simulink subsystem "MFTrailerTires"  (R2023a)
settings: Solver=VariableStepAuto  StartTime=0.0  StopTime=10.0  RelTol=1e-3
undefined symbols (not defined in the file): PlntTraInitVertPos, PlntTraNumWhlFrntAxl, PlntTraWhlInitAngVel, PlntTraWhlNomPress
libraries: autolibutils x2, sharedtransform x2, vehdynlibtire x1, vehdynlibtirecommon x1
settings Model: ModifiedByFormat=The MathWorks, Inc.  Creator=The MathWorks, Inc.  LastModifiedBy=The MathWorks, Inc.
settings OptimizationCC: ReuseModelBlockBuffer=off

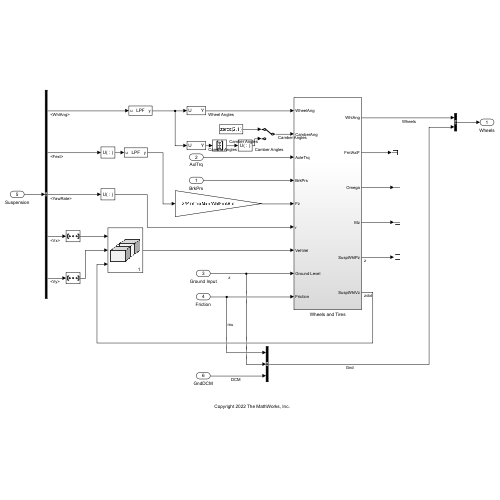
[thumbnail: Simulink's stored preview of the top-level diagram]
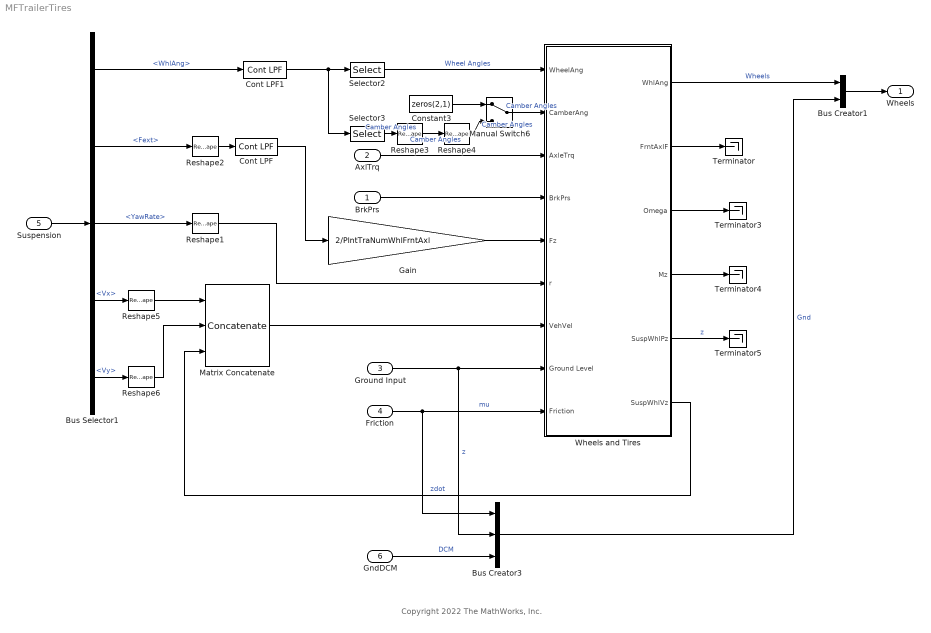
== system MFTrailerTires ==
  note: Copyright 2022 The MathWorks, Inc.
  BrkPrs : Inport
  AxlTrq : Inport  Port=2
  Ground Input : Inport  Port=3
  Friction : Inport  Port=4
  Suspension : Inport  Port=5
  GndDCM : Inport  Port=6
  Bus Creator1 : BusCreator  Inputs=2
  Bus Creator3 : BusCreator  Inputs=3
  Bus Selector1 : BusSelector  OutputSignals=Suspension.WhlAng,Suspension.Fext,Suspension.YawRate,Suspension.Vx,Suspension.Vy
  Constant3 : Constant  Value=zeros(2,1)  SampleTime=-1
  Cont LPF : autolibutils/Cont LPF  wc=100*2*pi  AbsoluteTolerance=auto  aMode=2
  Cont LPF1 : autolibutils/Cont LPF  wc=100*2*pi  AbsoluteTolerance=auto  aMode=2
  Gain : Gain  Gain=2/PlntTraNumWhlFrntAxl
  Manual Switch6 : ManualSwitch
  Matrix Concatenate : Concatenate  NumInputs=3  Mode=Multidimensional array
  Reshape1 : Reshape
  Reshape2 : Reshape
  Reshape3 : Reshape  OutputDimensionality=Column vector (2-D)
  Reshape4 : Reshape
  Reshape5 : Reshape  OutputDimensionality=Row vector (2-D)
  Reshape6 : Reshape  OutputDimensionality=Row vector (2-D)
  Selector2 : Selector  NumberOfDimensions=2  InputPortWidth=3  IndexOptions=Index vector (dialog),Select all  Indices=3,1  OutputSizes=1,1
  Selector3 : Selector  NumberOfDimensions=2  InputPortWidth=3  IndexOptions=Index vector (dialog),Select all  Indices=1,1  OutputSizes=1,1
  Terminator{,3..5} (4 alike) : Terminator
  Wheels and Tires : Subsystem  VariantControl=0
  Wheels : Outport  VectorParamsAs1DForOutWhenUnconnected=off
  wires:
  Ground Input/1 -> Wheels and Tires/8(Ground Level), Bus Creator3/2  "z"
  GndDCM/1 -> Bus Creator3/3  "DCM"
  Friction/1 -> Bus Creator3/1, Wheels and Tires/9(Friction)  "mu"
  Bus Creator3/1 -> Bus Creator1/2  "Gnd"
  Bus Creator1/1 -> Wheels/1
  Selector3/1 -> Reshape3/1  "Camber Angles"
  Reshape2/1 -> Cont LPF/1
  Reshape1/1 -> Wheels and Tires/6(r)
  Cont LPF/1 -> Gain/1
  BrkPrs/1 -> Wheels and Tires/4(BrkPrs)
  Cont LPF1/1 -> Selector3/1, Selector2/1
  Wheels and Tires/6(SuspWhlVz) -> Matrix Concatenate/3  "zdot"
  Bus Selector1/1 -> Cont LPF1/1  "<WhlAng>"
  Manual Switch6/1 -> Wheels and Tires/2(CamberAng)  "Camber Angles"
  Bus Selector1/5 -> Reshape6/1  "<Vy>"
  Bus Selector1/4 -> Reshape5/1  "<Vx>"
  Reshape3/1 -> Reshape4/1  "Camber Angles"
  Suspension/1 -> Bus Selector1/1
  Bus Selector1/3 -> Reshape1/1  "<YawRate>"
  Wheels and Tires/3(Omega) -> Terminator3/1
  Constant3/1 -> Manual Switch6/1
  Wheels and Tires/4(Mz) -> Terminator4/1
  Wheels and Tires/5(SuspWhlPz) -> Terminator5/1  "z"
  Bus Selector1/2 -> Reshape2/1  "<Fext>"
  AxlTrq/1 -> Wheels and Tires/3(AxleTrq)
  Reshape4/1 -> Manual Switch6/2  "Camber Angles"
  Wheels and Tires/1(WhlAng) -> Bus Creator1/1  "Wheels"
  Gain/1 -> Wheels and Tires/5(Fz)
  Selector2/1 -> Wheels and Tires/1(WheelAng)  "Wheel Angles"
  Matrix Concatenate/1 -> Wheels and Tires/7(VehVel)
  Wheels and Tires/2(FrntAxlF) -> Terminator/1
  Reshape5/1 -> Matrix Concatenate/1
  Reshape6/1 -> Matrix Concatenate/2

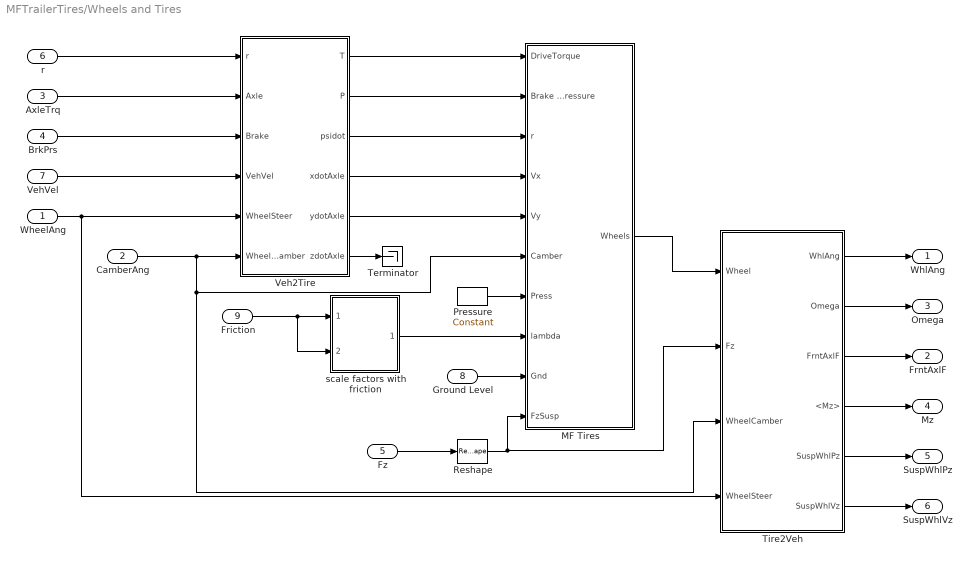
== system MFTrailerTires/Wheels and Tires ==
  WheelAng : Inport
  CamberAng : Inport  Port=2  Unit=rad
  AxleTrq : Inport  Port=3
  BrkPrs : Inport  Port=4
  Fz : Inport  Port=5  Unit=N
  r : Inport  Port=6
  VehVel : Inport  Port=7
  Ground Level : Inport  Port=8
  Friction : Inport  Port=9  Unit=1
  MF Tires : Subsystem  VariantControl=0
  Pressure : vehdynlibtirecommon/Constant  const=PlntTraWhlNomPress  numWheels=2
  Reshape : Reshape
  Terminator : Terminator
  Tire2Veh : Subsystem
  Veh2Tire : Subsystem
  scale factors with friction : Subsystem  mask{numWheels=6}
      mask prompts: numWheels "Number of wheels"
  WhlAng : Outport  VectorParamsAs1DForOutWhenUnconnected=off
  FrntAxlF : Outport  Port=2  Unit=N  VectorParamsAs1DForOutWhenUnconnected=off
  Omega : Outport  Port=3  VectorParamsAs1DForOutWhenUnconnected=off
  Mz : Outport  Port=4  Unit=N*m  VectorParamsAs1DForOutWhenUnconnected=off
  SuspWhlPz : Outport  Port=5  VectorParamsAs1DForOutWhenUnconnected=off
  SuspWhlVz : Outport  Port=6  VectorParamsAs1DForOutWhenUnconnected=off
  wires:
  Reshape/1 -> MF Tires/10(FzSusp), Tire2Veh/2(Fz)
  Ground Level/1 -> MF Tires/9(Gnd)
  Pressure/1 -> MF Tires/7(Press)
  scale factors with friction/1(lambdas) -> MF Tires/8(lambda)
  Fz/1 -> Reshape/1
  AxleTrq/1 -> Veh2Tire/2(Axle)
  BrkPrs/1 -> Veh2Tire/3(Brake)
  VehVel/1 -> Veh2Tire/4(VehVel)
  Veh2Tire/1(T) -> MF Tires/1(DriveTorque)
  Veh2Tire/2(P) -> MF Tires/2(Brake Pressure)
  Veh2Tire/4(xdotAxle) -> MF Tires/4(Vx)
  Veh2Tire/5(ydotAxle) -> MF Tires/5(Vy)
  Veh2Tire/3(psidot) -> MF Tires/3(r)
  MF Tires/1(Wheels) -> Tire2Veh/1(Wheel)
  WheelAng/1 -> Veh2Tire/5(WheelSteer), Tire2Veh/4(WheelSteer)
  Tire2Veh/2(Omega) -> Omega/1
  Tire2Veh/3(FrntAxlF) -> FrntAxlF/1
  Tire2Veh/4(<Mz>) -> Mz/1
  Friction/1 -> scale factors with friction/1(lamda_mu_x), scale factors with friction/2(lamda_mu_y)
  r/1 -> Veh2Tire/1(r)
  Veh2Tire/6(zdotAxle) -> Terminator/1
  Tire2Veh/5(SuspWhlPz) -> SuspWhlPz/1
  Tire2Veh/6(SuspWhlVz) -> SuspWhlVz/1
  CamberAng/1 -> MF Tires/6(Camber), Tire2Veh/3(WheelCamber), Veh2Tire/6(WheelCamber)
  Tire2Veh/1(WhlAng) -> WhlAng/1

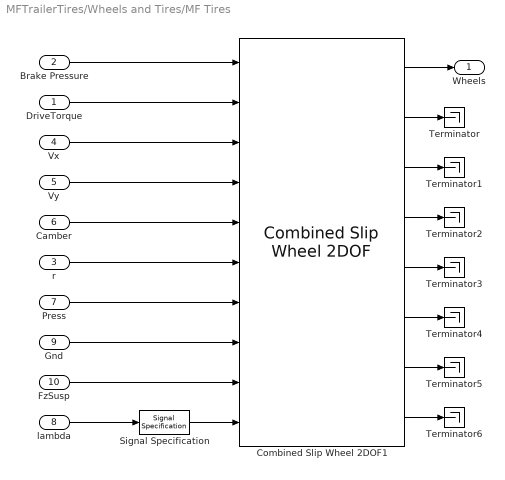
== system MFTrailerTires/Wheels and Tires/MF Tires ==
  DriveTorque : Inport
  Brake Pressure : Inport  Port=2
  r : Inport  Port=3
  Vx : Inport  Port=4
  Vy : Inport  Port=5
  Camber : Inport  Port=6
  Press : Inport  Port=7  Unit=Pa
  lambda : Inport  Port=8  Unit=1
  Gnd : Inport  Port=9
  FzSusp : Inport  Port=10
  Combined Slip Wheel 2DOF1 : vehdynlibtire/Combined Slip Wheel 2DOF  tireType=Mid-size passenger car 235/45R18  BrakeType=Disc  vertType=Magic Formula  plySteer=off  turnslip=off  mu_static=PlntTraBrkStcFricCffFrnt  mu_kinetic=PlntTraBrkKinFricCffFrnt  disk_abore=PlntTraBrkActrBoreFrnt  Rm=PlntTraBrkPadMeanRadiusFrnt  num_pads=PlntTraBrkNumPadsFrnt  drum_abore=0.0508  drum_a=0.123  drum_c=0.212  drum_r=0.15  drum_theta1=0  drum_theta2=126  brake_p_bpt=[1 11.4736842105263 21.9473684210526 32.4210526315789 42.8947368421053 53.3684210526316 63.8421052631579 74.3157894736842 84.7894736842105 95.2631578947368 105.736842105263 116.210526315789 126.684210526316 137.157894736842 147.631578947368 158.105263157895 168.578947368421 179.052631578947 189.526315789474 200]  brake_n_bpt=[0 52.6315789473684 105.263157894737 157.894736842105 210.526315789474 263.157894736842 315.789473684211 368.421052631579 421.052631578947 473.684210526316 526.315789473684 578.947368421053 631.578947368421 684.210526315789 736.842105263158 789.473684210526 842.105263157895 894.736842105263 947.368421052632 1000]  f_brake_t=[43.4900602404453 42.5056030554862 41.5350898940194 40.5780454442085 39.6340111501808 38.7025443887544 37.7832176914519 36.8756180088306 35.9793460143796 35.0940154454303 34.2192524787115 33.3546951383474 32.4999927342521 31.6548053290159 30.8188032315107 29.991666515561 29.1730845621415 28.362755623661 27.5603864089927 26.765691687993;498.991217495636 487.695866636631 476.560505099801 465.579679307235 454.748127933653 444.060772460445 433.51270824929 423.099196101319 412.81565427025 402.657650900201 392.620896861006 382.701238955775 372.894653477208 363.197240090814 353.605216024701 344.114910546964 334.722759712992 325.425301366216 316.219170376863 307.10109410434;954.492374750826 932.886130217776 911.585920305583 890.581313170261 869.862244717126 849.419000532136 829.242198807128 809.322774193808 789.651962526121 770.221286354971 751.0225412433 732.047782773203 713.289314220164 694.739674852612 676.391628817892 658.238154578366 640.272434863842 622.48784710877 604.877954344734 587.436496520688;1409.99353200602 1378.07639379892 1346.61133551136 1315.58294703329 1284.9763615006 1254.77722860383 1224.97168936497 1195.5463522863 1166.48827078199 1137.78492180974 1109.42418562559 1081.39432659063 1053.68397496312 1026.28210961441 999.178041611083 972.361398609768 945.822110014692 919.550392851325 893.536738312604 867.771898937035;1865.49468926121 1823.26665738007 1781.63675071715 1740.58458089631 1700.09047828407 1660.13545667552 1620.7011799228 1581.76993037878 1543.32457903786 1505.34855726451 1467.82583000789 1430.74087040806 1394.07863570608 1357.82454437621 1321.96445440427 1286.48464264117 1251.37178516554 1216.61293859388 1182.19552228048 1148.10730135338;2320.9958465164 2268.45692096121 2216.66216592293 2165.58621475934 2115.20459506754 2065.49368474721 2016.43067048064 1967.99350847127 1920.16088729373 1872.91219271928 1826.22747439018 1780.08741422549 1734.47329644903 1689.36697913801 1644.75086719747 1600.60788667257 1556.92146031639 1513.67548433643 1470.85430624835 1428.44270376973;2776.49700377159 2713.64718454235 2651.68758112871 2590.58784862237 2530.31871185102 2470.8519128189 2412.16016103848 2354.21708656376 2296.9971955496 2240.47582817405 2184.62911877248 2129.43395804292 2074.86795719199 2020.9094138998 1967.53727999066 1914.73113070398 1862.47113546724 1810.73803007899 1759.51309021622 1708.77810618608;3231.99816102678 3158.8374481235 3086.71299633449 3015.58948248539 2945.43282863449 2876.21014089059 2807.88965159632 2740.44066465625 2673.83350380547 2608.03946362882 2543.03076315477 2478.78050186034 2415.26261793494 2352.4518486616 2290.32369278385 2228.85437473538 2168.02081061809 2107.80057582154 2048.17187418409 1989.11350860242;3687.49931828197 3604.02771170464 3521.73841154027 3440.59111634842 3360.54694541796 3281.56836896228 3203.61914215416 3126.66424274874 3050.66981206134 2975.60309908359 2901.43240753707 2828.12704567777 2755.6572786779 2683.9942834234 2613.11010557704 2542.97761876678 2473.57048576894 2404.8631215641 2336.83065815196 2269.44891101877;4143.00047553716 4049.21797528579 3956.76382674606 3865.59275021144 3775.66106220143 3686.92659703397 3599.34863271199 3512.88782084123 3427.50612031721 3343.16673453836 3259.83405191936 3177.4735894952 3096.05193942085 3015.5367181852 2935.89651837023 2857.10086279818 2779.12016091979 2701.92566730665 2625.48944211983 2549.78431343512;4598.50163279235 4494.40823886693 4391.78924195184 4290.59438407447 4190.77517898491 4092.28482510566 3995.07812326983 3899.11139893372 3804.34242857308 3710.73036999313 3618.23569630166 3526.82013331263 3436.44660016381 3347.079152947 3258.68293116342 3171.22410682959 3084.66983607064 2998.98821304921 2914.1482260877 2830.11971585147;5054.00279004754 4939.59850244808 4826.81465715762 4715.59601793749 4605.88929576838 4497.64305317735 4390.80761382767 4285.3349770262 4181.17873682896 4078.2940054479 3976.63734068395 3876.16667713006 3776.84126090677 3678.62158770879 3581.46934395661 3485.34735086099 ...(+2764 chars)]  tireParamSet=C:\SimTemp\GCAPS_Goodyear_MarathonRSA_295_75_R22.5_8.25J_141L_MF62turnslip_CA_YL_MAY042020.tir  PRESMAX=PlntTraWhlMaxPress  PRESMIN=PlntTraWhlMinPress  FZMAX=PlntTraWhlMaxFz  FZMIN=PlntTraWhlMinFz  VXLOW=PlntTraWhlVelTolLowVel  KPUMAX=PlntTraWhlMaxSlipRatio  KPUMIN=PlntTraWhlMinSlipRatio  ALPMAX=PlntTraWhlMaxSlipAngle  ALPMIN=PlntTraWhlMinSlipAngle  CAMMAX=PlntTraWhlMaxCmbr  CAMMIN=PlntTraWhlMinCmbr  LONGVL=PlntTraWhlLongSpd  FxRelFreqLwrLim=200*pi  FyRelFreqLwrLim=200*pi  MyRelFreqLwrLim=100*pi  omegao=[PlntTraWhlInitAngVel PlntTraWhlInitAngVel]  br=PlntTraWhlDampCoeff  UNLOADED_RADIUS=PlntTraWhlUnldRadius  NOMPRES=PlntTraWhlNomPress  FNOMIN=PlntTraWhlNomNorlForce  WIDTH=PlntTraWhlWidth  RIM_RADIUS=PlntTraWhlRimRadius  MASS=PlntTraWhlMass  IYY=PlntTraWhlInertia  GRAVITY=-9.81  zo=-PlntTraInitVertPos  zdoto=0  BREFF=8.392  DREFF=0.03576  FREFF=0.4661  Q_RE0=1.0016  Q_V1=0.0003732  Q_V2=0.02362  Q_FZ1=0  Q_FZ2=133.78  Q_FZ3=0  Q_FCX=0  Q_FCY=0  Q_FCY2=0  PFZ1=0  VERTICAL_STIFFNESS=910293.6  VERTICAL_DAMPING=PlntTraWhlVertDampCoeff  BOTTOM_OFFST=0.01  BOTTOM_STIFF=2000000  LONGITUDINAL_STIFFNESS=658043.3  LATERAL_STIFFNESS=334950.6  PCFX1=-0.05681  PCFX2=0  PCFX3=0  PCFY1=-0.012727  PCFY2=0  PCFY3=0  Q_RA1=1  Q_RA2=0.167  Q_RB1=1.4176  Q_RB2=-3.104  PCX1=1.6344  PDX1=0.8142  PDX2=-0.16106  PDX3=0  PEX1=0.14852  PEX2=0.10924  PEX3=0  PEX4=0.6315  PKX1=12.27  PKX2=0.07478  PKX3=-0.02593  PHX1=-0.002517  PHX2=-5.505e-05  PVX1=0.018635  PVX2=0.004217  PPX1=0  PPX2=0  PPX3=0  PPX4=0  RBX1=14.568  RBX2=26.13  RBX3=0  RCX1=0.67  REX1=-10  REX2=1.2903  RHX1=0.006853  QSX1=0.0015863  QSX2=0.7911  QSX3=0.005838  QSX4=0.6123  QSX5=1.0173  QSX6=1.0795  QSX7=-1  QSX8=-0.07876  QSX9=1.5937  QSX10=0.20124  QSX11=7.712  QSX12=0  QSX13=0  QSX14=0  PPMX1=0  PCY1=1.7918  PDY1=0.8339  PDY2=-0.16352  PDY3=0  PEY1=0.3527  PEY2=-0.4847  PEY3=-0.04566  PEY4=-0.8786  PEY5=0  PKY1=-25.044  PKY2=5  PKY3=-0.35276  PKY4=1.397  PKY5=0  PKY6=-0.14207  PKY7=0.2761  PHY1=0.004573  PHY2=0.0011903  PVY1=0.012717  PVY2=-0.005622  PVY3=-0.5051  PVY4=-0.20847  PPY1=0  PPY2=0  PPY3=0  PPY4=0  PPY5=0  RBY1=11.94  RBY2=7.527  RBY3=-0.04993  RBY4=0  RCY1=1.011  REY1=0.5603  REY2=-0.015398  RHY1=0.003565  RHY2=-0.004565  RVY1=-0.02114  RVY2=0.00636  RVY3=0.5299  RVY4=15  RVY5=2.2  RVY6=6.517  QSY1=0.01  QSY2=0  QSY3=0.0004  QSY4=4e-05  QSY5=0  QSY6=0  QSY7=0.85  QSY8=-0.4  QBZ1=5  QBZ2=0.11227  QBZ3=0  QBZ4=0.3959  QBZ5=0.6941  QBZ6=0  QBZ9=7.076  QBZ10=0  QCZ1=1.6  QDZ1=0.05489  QDZ2=-0.014706  QDZ3=0.23333  QDZ4=0  QDZ6=-0.002125  QDZ7=0.0019598  QDZ8=-0.05395  QDZ9=0.011456  QDZ10=0  QDZ11=0  QEZ1=-0.2972  QEZ2=0.0005504  QEZ3=0  QEZ4=0.8904  QEZ5=-15  QHZ1=0.009102  QHZ2=-0.0012268  QHZ3=0.24217  QHZ4=-0.2619  PPZ1=0  PPZ2=0  SSZ1=-0.011962  SSZ2=0.01055  SSZ3=0.885  SSZ4=-0.3521  PDXP1=0.4  PDXP2=0  PDXP3=0  PKYP1=0.1  PDYP1=0.4  PDYP2=0  PDYP3=0  PDYP4=0  PHYP1=1  PHYP2=0.15  PHYP3=0  PHYP4=-4  PECP1=0.68093  PECP2=1.5779e-08  QDTP1=5.6762  QCRP1=0.11047  QCRP2=0.1  QBRP1=0.10576  QDRP1=1  QDRP2=0  aMode=2
      settings: SourceProductName=Vehicle Dynamics Blockset
  Signal Specification : SignalSpecification  Unit=1
  Terminator{,1..6} (7 alike) : Terminator
  Wheels : Outport  VectorParamsAs1DForOutWhenUnconnected=off
  wires:
  FzSusp/1 -> Combined Slip Wheel 2DOF1/9
  Combined Slip Wheel 2DOF1/2 -> Terminator/1
  Gnd/1 -> Combined Slip Wheel 2DOF1/8
  Combined Slip Wheel 2DOF1/1 -> Wheels/1
  Brake Pressure/1 -> Combined Slip Wheel 2DOF1/1
  DriveTorque/1 -> Combined Slip Wheel 2DOF1/2
  Press/1 -> Combined Slip Wheel 2DOF1/7
  r/1 -> Combined Slip Wheel 2DOF1/6
  Camber/1 -> Combined Slip Wheel 2DOF1/5
  lambda/1 -> Signal Specification/1
  Vx/1 -> Combined Slip Wheel 2DOF1/3
  Vy/1 -> Combined Slip Wheel 2DOF1/4
  Signal Specification/1 -> Combined Slip Wheel 2DOF1/10
  Combined Slip Wheel 2DOF1/3 -> Terminator1/1
  Combined Slip Wheel 2DOF1/4 -> Terminator2/1
  Combined Slip Wheel 2DOF1/7 -> Terminator5/1
  Combined Slip Wheel 2DOF1/6 -> Terminator4/1
  Combined Slip Wheel 2DOF1/5 -> Terminator3/1
  Combined Slip Wheel 2DOF1/8 -> Terminator6/1

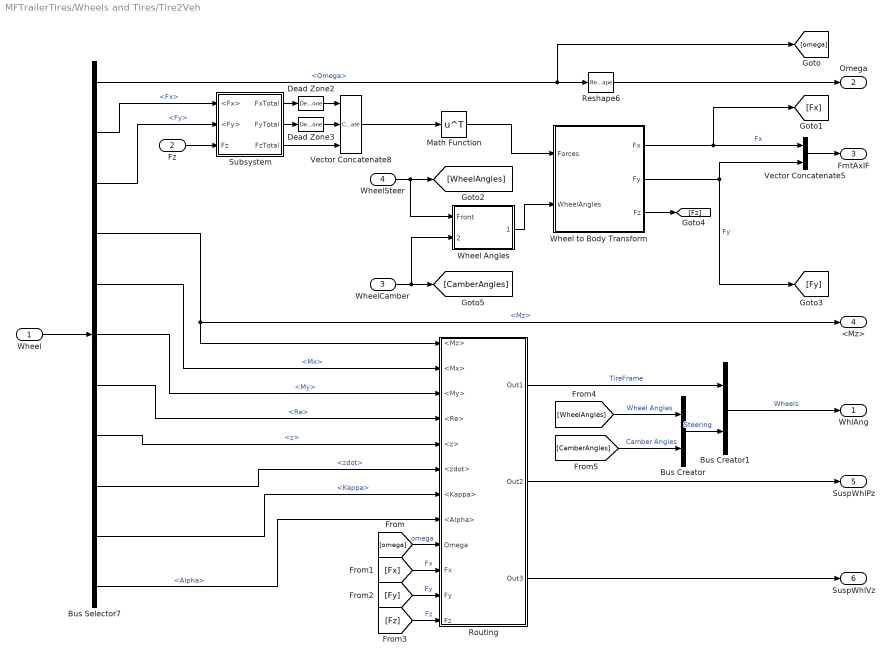
== system MFTrailerTires/Wheels and Tires/Tire2Veh ==
  Wheel : Inport
  Fz : Inport  Port=2
  WheelCamber : Inport  Port=3
  WheelSteer : Inport  Port=4
  Bus Creator : BusCreator  Inputs=2
  Bus Creator1 : BusCreator  Inputs=2
  Bus Selector7 : BusSelector  OutputSignals=Omega,Fx,Fy,Mz,Mx,My,Re,z,zdot,Kappa,Alpha
  Dead Zone2 : DeadZone  LowerValue=-5  UpperValue=5  ZeroCross=off
  Dead Zone3 : DeadZone  LowerValue=-10  UpperValue=10  ZeroCross=off
  Math Function : Math  Operator=transpose  SignedPower=on
  Reshape6 : Reshape  OutputDimensionality=Customize  OutputDimensions=[2,1]
  Routing : Subsystem
  Subsystem : Subsystem
  Vector Concatenate5 : Concatenate  Mode=Multidimensional array  ConcatenateDimension=2
  Vector Concatenate8 : Concatenate  NumInputs=3  Mode=Multidimensional array  ConcatenateDimension=2
  Wheel Angles : Subsystem
  Wheel to Body Transform : Subsystem
  WhlAng : Outport  VectorParamsAs1DForOutWhenUnconnected=off
  Omega : Outport  Port=2  VectorParamsAs1DForOutWhenUnconnected=off
  FrntAxlF : Outport  Port=3  VectorParamsAs1DForOutWhenUnconnected=off
  <Mz> : Outport  Port=4  VectorParamsAs1DForOutWhenUnconnected=off
  SuspWhlPz : Outport  Port=5  VectorParamsAs1DForOutWhenUnconnected=off
  SuspWhlVz : Outport  Port=6  VectorParamsAs1DForOutWhenUnconnected=off
  wires:
  Dead Zone3/1 -> Vector Concatenate8/2
  Dead Zone2/1 -> Vector Concatenate8/1
  Subsystem/3(FzTotal) -> Vector Concatenate8/3
  Subsystem/2(FyTotal) -> Dead Zone3/1
  Subsystem/1(FxTotal) -> Dead Zone2/1
  Fz/1 -> Subsystem/3(Fz)
  Bus Selector7/3 -> Subsystem/2(<Fy>)  "<Fy>"
  Bus Selector7/2 -> Subsystem/1(<Fx>)  "<Fx>"
  Vector Concatenate8/1 -> Math Function/1
  Math Function/1 -> Wheel to Body Transform/1(Forces)
  Wheel to Body Transform/1(Fx) -> Vector Concatenate5/1, [Fx]  "Fx"
  Vector Concatenate5/1 -> FrntAxlF/1
  Wheel/1 -> Bus Selector7/1
  Reshape6/1 -> Omega/1
  Wheel to Body Transform/2(Fy) -> Vector Concatenate5/2, [Fy]  "Fy"
  Wheel Angles/1(Vehicle) -> Wheel to Body Transform/2(WheelAngles)
  Bus Selector7/1 -> [omega], Reshape6/1  "<Omega>"
  WheelSteer/1 -> Wheel Angles/1(Front), [WheelAngles]
  Bus Selector7/4 -> <Mz>/1, Routing/1(<Mz>)  "<Mz>"
  Wheel to Body Transform/3(Fz) -> [Fz]
  WheelCamber/1 -> Wheel Angles/2(Camber), [CamberAngles]
  Bus Selector7/5 -> Routing/2(<Mx>)  "<Mx>"
  Bus Selector7/6 -> Routing/3(<My>)  "<My>"
  Bus Selector7/7 -> Routing/4(<Re>)  "<Re>"
  [omega] -> Routing/9(Omega)  "omega"
  [Fx] -> Routing/10(Fx)  "Fx"
  Bus Selector7/8 -> Routing/5(<z>)  "<z>"
  [Fy] -> Routing/11(Fy)  "Fy"
  [Fz] -> Routing/12(Fz)  "Fz"
  Bus Selector7/9 -> Routing/6(<zdot>)  "<zdot>"
  Bus Selector7/10 -> Routing/7(<Kappa>)  "<Kappa>"
  Routing/2(Out2) -> SuspWhlPz/1
  Routing/3(Out3) -> SuspWhlVz/1
  [WheelAngles] -> Bus Creator/1  "Wheel Angles"
  Bus Creator1/1 -> WhlAng/1  "Wheels"
  Routing/1(Out1) -> Bus Creator1/1  "TireFrame"
  [CamberAngles] -> Bus Creator/2  "Camber Angles"
  Bus Creator/1 -> Bus Creator1/2  "Steering"
  Bus Selector7/11 -> Routing/8(<Alpha>)  "<Alpha>"

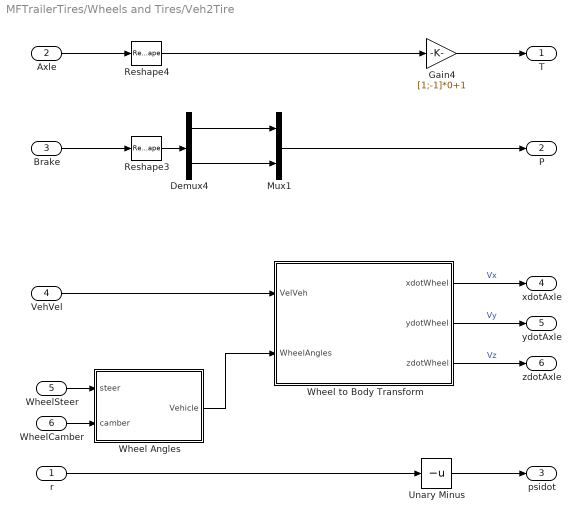
== system MFTrailerTires/Wheels and Tires/Veh2Tire ==
  r : Inport
  Axle : Inport  Port=2
  Brake : Inport  Port=3
  VehVel : Inport  Port=4
  WheelSteer : Inport  Port=5
  WheelCamber : Inport  Port=6
  Demux4 : Demux  Outputs=2
  Gain4 : Gain  Gain=[1;-1]*0+1
  Mux1 : Mux  Inputs=2
  Reshape3 : Reshape
  Reshape4 : Reshape
  Unary Minus : UnaryMinus
  Wheel Angles : Subsystem
  Wheel to Body Transform : Subsystem
  T : Outport  Unit=N*m  VectorParamsAs1DForOutWhenUnconnected=off
  P : Outport  Port=2  Unit=Pa  VectorParamsAs1DForOutWhenUnconnected=off
  psidot : Outport  Port=3  Unit=rad/s  VectorParamsAs1DForOutWhenUnconnected=off
  xdotAxle : Outport  Port=4  Unit=m/s  VectorParamsAs1DForOutWhenUnconnected=off
  ydotAxle : Outport  Port=5  Unit=m/s  VectorParamsAs1DForOutWhenUnconnected=off
  zdotAxle : Outport  Port=6  Unit=m/s  VectorParamsAs1DForOutWhenUnconnected=off
  wires:
  Demux4/2 -> Mux1/2
  Demux4/1 -> Mux1/1
  Brake/1 -> Reshape3/1
  Axle/1 -> Reshape4/1
  Wheel to Body Transform/1(xdotWheel) -> xdotAxle/1  "Vx"
  Wheel to Body Transform/2(ydotWheel) -> ydotAxle/1  "Vy"
  WheelSteer/1 -> Wheel Angles/1(steer)
  Mux1/1 -> P/1
  r/1 -> Unary Minus/1
  Reshape3/1 -> Demux4/1
  Gain4/1 -> T/1
  Reshape4/1 -> Gain4/1
  VehVel/1 -> Wheel to Body Transform/1(VelVeh)
  Wheel to Body Transform/3(zdotWheel) -> zdotAxle/1  "Vz"
  WheelCamber/1 -> Wheel Angles/2(camber)
  Unary Minus/1 -> psidot/1
  Wheel Angles/1(Vehicle) -> Wheel to Body Transform/2(WheelAngles)

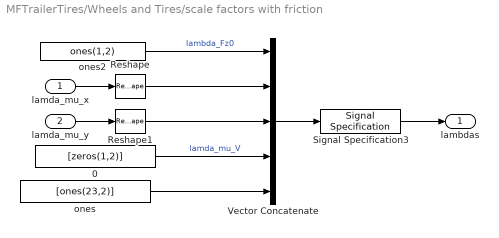
== system MFTrailerTires/Wheels and Tires/scale factors with friction ==
  lamda_mu_x : Inport
  lamda_mu_y : Inport  Port=2
  0 : Constant  Value=[zeros(1,2)]  VectorParams1D=off
  Reshape : Reshape  OutputDimensionality=Row vector (2-D)  OutputDimensions=[1,numWheels]
  Reshape1 : Reshape  OutputDimensionality=Row vector (2-D)  OutputDimensions=[1,numWheels]
  Signal Specification3 : SignalSpecification  Unit=1
  Vector Concatenate : Concatenate  NumInputs=5  Mode=Multidimensional array
  ones : Constant  Value=[ones(23,2)]  VectorParams1D=off
  ones2 : Constant  Value=ones(1,2)  VectorParams1D=off
  lambdas : Outport  Unit=1  VectorParamsAs1DForOutWhenUnconnected=off
  wires:
  Signal Specification3/1 -> lambdas/1
  Reshape/1 -> Vector Concatenate/2
  Reshape1/1 -> Vector Concatenate/3
  0/1 -> Vector Concatenate/4  "lamda_mu_V"
  ones/1 -> Vector Concatenate/5
  Vector Concatenate/1 -> Signal Specification3/1
  ones2/1 -> Vector Concatenate/1  "lambda_Fz0"
  lamda_mu_x/1 -> Reshape/1
  lamda_mu_y/1 -> Reshape1/1

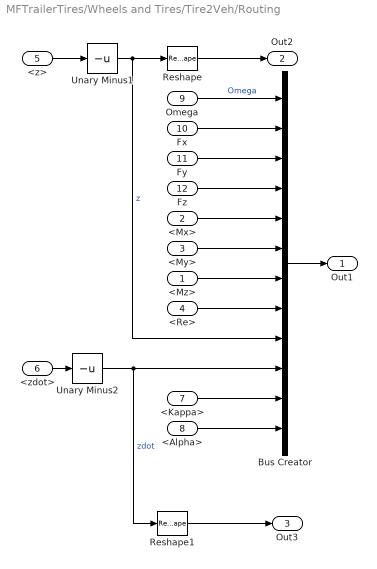
== system MFTrailerTires/Wheels and Tires/Tire2Veh/Routing ==
  <Mz> : Inport
  <Mx> : Inport  Port=2
  <My> : Inport  Port=3
  <Re> : Inport  Port=4
  <z> : Inport  Port=5
  <zdot> : Inport  Port=6
  <Kappa> : Inport  Port=7
  <Alpha> : Inport  Port=8
  Omega : Inport  Port=9
  Fx : Inport  Port=10
  Fy : Inport  Port=11
  Fz : Inport  Port=12
  Bus Creator : BusCreator  Inputs=12
  Reshape : Reshape  OutputDimensionality=Row vector (2-D)
  Reshape1 : Reshape  OutputDimensionality=Row vector (2-D)
  Unary Minus1 : UnaryMinus
  Unary Minus2 : UnaryMinus
  Out1 : Outport  VectorParamsAs1DForOutWhenUnconnected=off
  Out2 : Outport  Port=2  VectorParamsAs1DForOutWhenUnconnected=off
  Out3 : Outport  Port=3  VectorParamsAs1DForOutWhenUnconnected=off
  wires:
  <Re>/1 -> Bus Creator/8
  Unary Minus1/1 -> Reshape/1, Bus Creator/9  "z"
  Fz/1 -> Bus Creator/4
  <zdot>/1 -> Unary Minus2/1
  <Mz>/1 -> Bus Creator/7
  Unary Minus2/1 -> Reshape1/1, Bus Creator/10  "zdot"
  <z>/1 -> Unary Minus1/1
  Bus Creator/1 -> Out1/1
  Fy/1 -> Bus Creator/3
  Omega/1 -> Bus Creator/1  "Omega"
  Fx/1 -> Bus Creator/2
  Reshape1/1 -> Out3/1
  <Kappa>/1 -> Bus Creator/11
  Reshape/1 -> Out2/1
  <Mx>/1 -> Bus Creator/5
  <My>/1 -> Bus Creator/6
  <Alpha>/1 -> Bus Creator/12

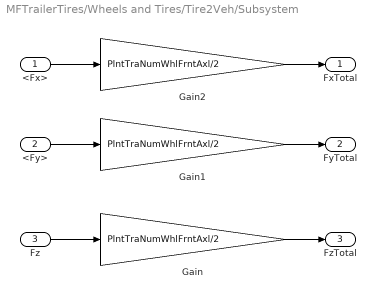
== system MFTrailerTires/Wheels and Tires/Tire2Veh/Subsystem ==
  <Fx> : Inport
  <Fy> : Inport  Port=2
  Fz : Inport  Port=3
  Gain : Gain  Gain=PlntTraNumWhlFrntAxl/2
  Gain1 : Gain  Gain=PlntTraNumWhlFrntAxl/2
  Gain2 : Gain  Gain=PlntTraNumWhlFrntAxl/2
  FxTotal : Outport
  FyTotal : Outport  Port=2
  FzTotal : Outport  Port=3
  wires:
  Gain1/1 -> FyTotal/1
  <Fy>/1 -> Gain1/1
  Gain2/1 -> FxTotal/1
  Gain/1 -> FzTotal/1
  Fz/1 -> Gain/1
  <Fx>/1 -> Gain2/1

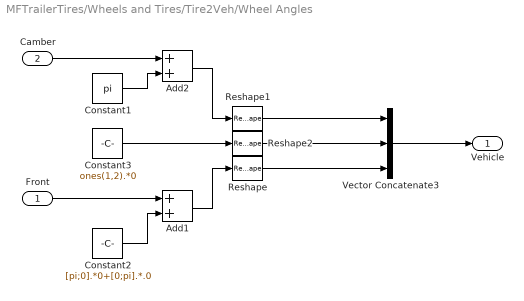
== system MFTrailerTires/Wheels and Tires/Tire2Veh/Wheel Angles ==
  Front : Inport
  Camber : Inport  Port=2
  Add1 : Sum
  Add2 : Sum
  Constant1 : Constant  Value=pi  SampleTime=-1
  Constant2 : Constant  Value=[pi;0].*0+[0;pi].*.0  SampleTime=-1
  Constant3 : Constant  Value=ones(1,2).*0  SampleTime=-1
  Reshape : Reshape  OutputDimensionality=Row vector (2-D)
  Reshape1 : Reshape  OutputDimensionality=Row vector (2-D)
  Reshape2 : Reshape  OutputDimensionality=Row vector (2-D)
  Vector Concatenate3 : Concatenate  NumInputs=3  Mode=Multidimensional array
  Vehicle : Outport  VectorParamsAs1DForOutWhenUnconnected=off
  wires:
  Reshape/1 -> Vector Concatenate3/3
  Reshape2/1 -> Vector Concatenate3/2
  Vector Concatenate3/1 -> Vehicle/1
  Constant2/1 -> Add1/2
  Front/1 -> Add1/1
  Reshape1/1 -> Vector Concatenate3/1
  Constant3/1 -> Reshape2/1
  Add1/1 -> Reshape/1
  Camber/1 -> Add2/1
  Add2/1 -> Reshape1/1
  Constant1/1 -> Add2/2

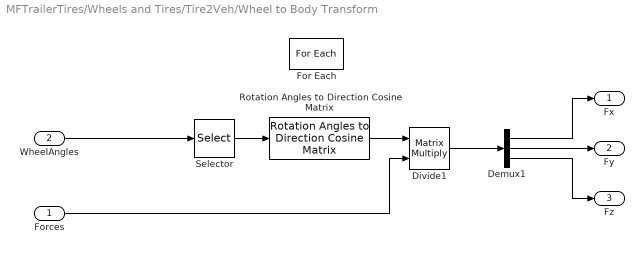
== system MFTrailerTires/Wheels and Tires/Tire2Veh/Wheel to Body Transform ==
  Forces : Inport  PortDimensions=[3,1]  Partition=on  PartitionDimension=2  PartitionWidth=1  PartitionOffset=0
  WheelAngles : Inport  Port=2  PortDimensions=[3,1]  Partition=on  PartitionDimension=2  PartitionWidth=1  PartitionOffset=0
  Demux1 : Demux  Outputs=3
  Divide1 : Product  Inputs=**  Multiplication=Matrix(*)
  For Each : ForEach  DisableCoverage=on
  Rotation Angles to Direction Cosine Matrix : sharedtransform/Rotation Angles to Direction Cosine Matrix  rotationOrder=ZYX  aMode=2
  Selector : Selector  InputPortWidth=3  IndexOptions=Index vector (dialog)  Indices=[3 2 1]  OutputSizes=1
  Fx : Outport  ConcatenationDimension=1  VectorParamsAs1DForOutWhenUnconnected=off
  Fy : Outport  Port=2  ConcatenationDimension=1  VectorParamsAs1DForOutWhenUnconnected=off
  Fz : Outport  Port=3  ConcatenationDimension=1  VectorParamsAs1DForOutWhenUnconnected=off
  wires:
  Divide1/1 -> Demux1/1
  Demux1/1 -> Fx/1
  Demux1/2 -> Fy/1
  Demux1/3 -> Fz/1
  Rotation Angles to Direction Cosine Matrix/1 -> Divide1/1
  Forces/1 -> Divide1/2
  WheelAngles/1 -> Selector/1
  Selector/1 -> Rotation Angles to Direction Cosine Matrix/1

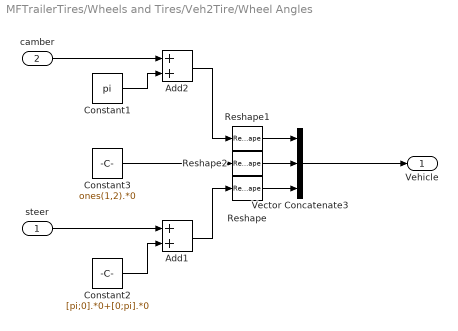
== system MFTrailerTires/Wheels and Tires/Veh2Tire/Wheel Angles ==
  steer : Inport
  camber : Inport  Port=2
  Add1 : Sum
  Add2 : Sum
  Constant1 : Constant  Value=pi  SampleTime=-1
  Constant2 : Constant  Value=[pi;0].*0+[0;pi].*0  SampleTime=-1
  Constant3 : Constant  Value=ones(1,2).*0  SampleTime=-1
  Reshape : Reshape  OutputDimensionality=Row vector (2-D)
  Reshape1 : Reshape  OutputDimensionality=Row vector (2-D)
  Reshape2 : Reshape  OutputDimensionality=Row vector (2-D)
  Vector Concatenate3 : Concatenate  NumInputs=3  Mode=Multidimensional array
  Vehicle : Outport  VectorParamsAs1DForOutWhenUnconnected=off
  wires:
  Constant2/1 -> Add1/2
  Constant3/1 -> Reshape2/1
  Vector Concatenate3/1 -> Vehicle/1
  Reshape/1 -> Vector Concatenate3/3
  Reshape1/1 -> Vector Concatenate3/1
  camber/1 -> Add2/1
  Reshape2/1 -> Vector Concatenate3/2
  steer/1 -> Add1/1
  Add1/1 -> Reshape/1
  Constant1/1 -> Add2/2
  Add2/1 -> Reshape1/1

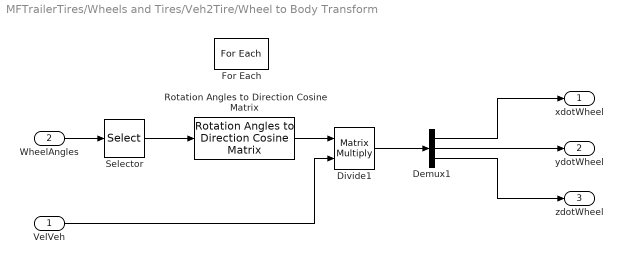
== system MFTrailerTires/Wheels and Tires/Veh2Tire/Wheel to Body Transform ==
  VelVeh : Inport  Partition=on  PartitionDimension=2  PartitionWidth=1  PartitionOffset=0
  WheelAngles : Inport  Port=2  Partition=on  PartitionDimension=2  PartitionWidth=1  PartitionOffset=0
  Demux1 : Demux  Outputs=3
  Divide1 : Product  Inputs=**  Multiplication=Matrix(*)
  For Each : ForEach  DisableCoverage=on
  Rotation Angles to Direction Cosine Matrix : sharedtransform/Rotation Angles to Direction Cosine Matrix  rotationOrder=ZYX  aMode=2
  Selector : Selector  InputPortWidth=3  IndexOptions=Index vector (dialog)  Indices=[3 2 1]  OutputSizes=1
  xdotWheel : Outport  ConcatenationDimension=1  VectorParamsAs1DForOutWhenUnconnected=off
  ydotWheel : Outport  Port=2  ConcatenationDimension=1  VectorParamsAs1DForOutWhenUnconnected=off
  zdotWheel : Outport  Port=3  ConcatenationDimension=1  VectorParamsAs1DForOutWhenUnconnected=off
  wires:
  Divide1/1 -> Demux1/1
  Demux1/1 -> xdotWheel/1
  Demux1/2 -> ydotWheel/1
  Demux1/3 -> zdotWheel/1
  Rotation Angles to Direction Cosine Matrix/1 -> Divide1/1
  VelVeh/1 -> Divide1/2
  WheelAngles/1 -> Selector/1
  Selector/1 -> Rotation Angles to Direction Cosine Matrix/1
